simulink model "Calculator"  (R2018a)
settings: Solver=VariableStepAuto  StartTime=0.0  StopTime=10.0  RelTol=1e-3  EnableMultiTasking=on
settings Model: Creator=LEGION  LastModifiedBy=user
settings OptimizationCC: LifeSpan=inf
settings DebuggingCC: SFUnexpectedBacktrackingDiag=warning  SFNoUnconditionalDefaultTransitionDiag=warning  SFExecutionAtInitializationDiag=none
settings CodeAppCC: StateflowObjectComments=on
settings GRTTargetCC: TargetLangStandard=C89/C90 (ANSI)  GeneratePreprocessorConditionals=Disable all
settings ConfigComp: CovMetricSettings=dw  CovHtmlReporting=on  CovSaveCumulativeToWorkspaceVar=on  CovSaveSingleToWorkspaceVar=on  CovExternalEMLEnable=off

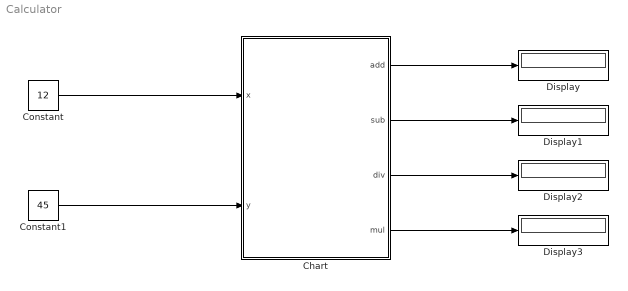
== system Calculator ==
  Chart : Stateflow chart  TreatAsAtomicUnit=on
  Constant : Constant  Value=12
  Constant1 : Constant  Value=45
  Display{,1..3} (4 alike) : Display
  wires:
  Chart/1(add) -> Display/1
  Chart/2(sub) -> Display1/1
  Chart/3(div) -> Display2/1
  Chart/4(mul) -> Display3/1
  Constant/1 -> Chart/1(x)
  Constant1/1 -> Chart/2(y)

== stateflow chart Calculator/Chart ==
  state Calculator_
    entry:
    add = x+y;
    sub = x-y;
    div = x/y;
    mul =x*y;
  (default) -> Calculator_
  data: x input; y input; add output; sub output; div output; mul output
